simulink model "lab_5"  (Simulink 7.3)
settings: Solver=ode3  StartTime=0.0  StopTime=500  FixedStep=0.001  RelTol=1e-3
settings Model: Creator=torres.g  LastModifiedBy=torres.g

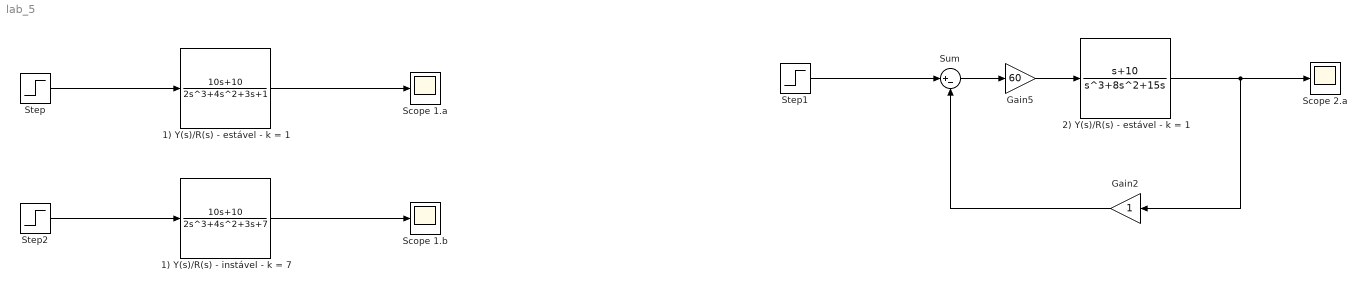
== system lab_5 ==
  1) Y(s)/R(s) - estável - k = 1 : TransferFcn  Numerator=[10 10]  Denominator=[2 4 3 1]
  1) Y(s)/R(s) - instável - k = 7 : TransferFcn  Numerator=[10 10]  Denominator=[2 4 3 7]
  2) Y(s)/R(s) - estável - k = 1 : TransferFcn  Numerator=[1 10]  Denominator=[1 8 15 0]
  Gain2 : Gain  ParameterDataType=fixdt(1, 16)  ParameterScaling=2^0  OutDataType=fixdt(1, 16)  OutScaling=2^0
  Gain5 : Gain  Gain=60  ParameterDataType=fixdt(1, 16)  ParameterScaling=2^0  OutDataType=fixdt(1, 16)  OutScaling=2^0
  Scope 1.a : Scope
  Scope 1.b : Scope
      settings: SaveName=ScopeData2
  Scope 2.a : Scope
  Step : Step  Time=0  SampleTime=0
  Step1 : Step  Time=0  SampleTime=0
  Step2 : Step  Time=0  SampleTime=0
  Sum : Sum  Inputs=|+-  OutDataType=fixdt(1, 16)  OutScaling=2^0
  wires:
  Step/1 -> 1) Y(s)/R(s) - estável - k = 1/1
  1) Y(s)/R(s) - estável - k = 1/1 -> Scope 1.a/1
  2) Y(s)/R(s) - estável - k = 1/1 -> Scope 2.a/1, Gain2/1
  Step2/1 -> 1) Y(s)/R(s) - instável - k = 7/1
  1) Y(s)/R(s) - instável - k = 7/1 -> Scope 1.b/1
  Gain2/1 -> Sum/2
  Step1/1 -> Sum/1
  Sum/1 -> Gain5/1
  Gain5/1 -> 2) Y(s)/R(s) - estável - k = 1/1
